simulink model "Task4_1"  (R2014a)
settings: Solver=ode45  StartTime=0.0  StopTime=10  RelTol=1e-3
values from neighbouring files (symbols this model uses):
  c = 0.15    [Task4.m]
  g = 9.81    [Task4.m]
  l = 2.5    [Task4.m]
  m = 0.75    [Task4.m]
settings Model: Creator=Eduardo  LastModifiedBy=Eduardo

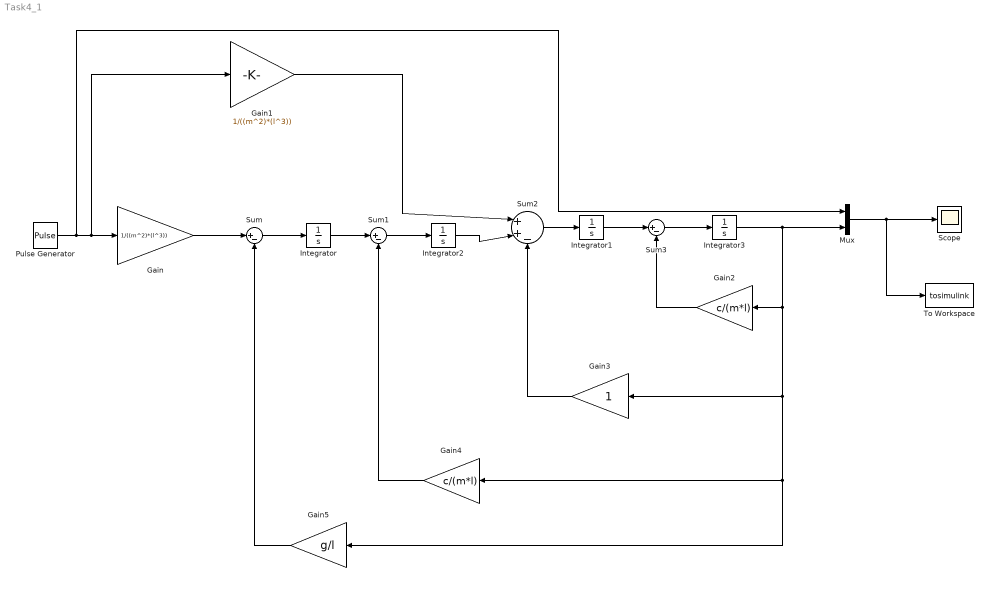
== system Task4_1 ==
  Gain : Gain  Gain=1/((m^2)*(l^3))
  Gain1 : Gain  Gain=1/((m^2)*(l^3))
  Gain2 : Gain  Gain=c/(m*l)
  Gain3 : Gain
  Gain4 : Gain  Gain=c/(m*l)
  Gain5 : Gain  Gain=g/l
  Integrator{,1..3} (4 alike) : Integrator
  Mux : Mux  Inputs=2
  Pulse Generator : DiscretePulseGenerator  PulseType=Time based  Amplitude=20  Period=100  PulseWidth=0.1
  Scope : Scope
  Sum : Sum  Inputs=|+-
  Sum1 : Sum  Inputs=|+-
  Sum2 : Sum  Inputs=|++-
  Sum3 : Sum  Inputs=|+-
  To Workspace : ToWorkspace  VariableName=tosimulink  SaveFormat=Timeseries  SampleTime=-1
  wires:
  Pulse Generator/1 -> Mux/1, Gain1/1, Gain/1
  Gain/1 -> Sum/1
  Sum/1 -> Integrator/1
  Integrator/1 -> Sum1/1
  Sum1/1 -> Integrator2/1
  Integrator2/1 -> Sum2/2
  Gain1/1 -> Sum2/1
  Sum2/1 -> Integrator1/1
  Integrator1/1 -> Sum3/1
  Sum3/1 -> Integrator3/1
  Integrator3/1 -> Mux/2, Gain5/1, Gain4/1, Gain3/1, Gain2/1
  Gain2/1 -> Sum3/2
  Gain3/1 -> Sum2/3
  Gain4/1 -> Sum1/2
  Gain5/1 -> Sum/2
  Mux/1 -> To Workspace/1, Scope/1
